simulink model "temp_gen_pch"  (Simulink 6.4)
settings: Solver=ode4  StartTime=0.0  StopTime=45  FixedStep=0.01  RelTol=1e-3
settings Model: Creator=oravec  LastModifiedBy=oravec
settings DataIOCC: LimitDataPoints=off  SignalLoggingName=sigsOut
settings OptimizationCC: InitFltsAndDblsToZero=off
settings DebuggingCC: SolverPrmCheckMsg=none  StrictBusMsg=None
settings HardwareCC: TargetHWDeviceType=32-bit Generic  TargetUnknown=on  ProdEqTarget=off

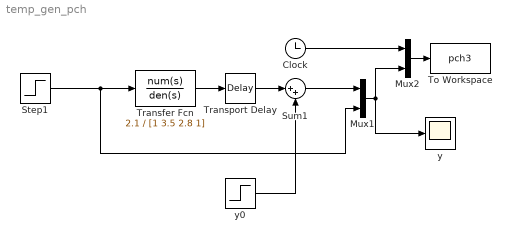
== system temp_gen_pch ==
  Clock : Clock
      settings: Decimation=10
  Mux1 : Mux  Inputs=2
  Mux2 : Mux  Inputs=2
  Step1 : Step  Time=0  Before=-1  After=2  SampleTime=0
  Sum1 : Sum  Inputs=|++
  To Workspace : ToWorkspace  VariableName=pch3  SampleTime=-1  SaveFormat=Array
  Transfer Fcn : TransferFcn  Numerator=2.1  Denominator=[1 3.5 2.8 1]
  Transport Delay : TransportDelay  DelayTime=0.3
  y : Scope
      settings: SaveName=ScopeData2
  y0 : Step  Time=0  After=3  SampleTime=0
  wires:
  Transfer Fcn/1 -> Transport Delay/1
  Mux1/1 -> y/1, Mux2/2
  Transport Delay/1 -> Sum1/1
  y0/1 -> Sum1/2
  Mux2/1 -> To Workspace/1
  Sum1/1 -> Mux1/1
  Clock/1 -> Mux2/1
  Step1/1 -> Transfer Fcn/1, Mux1/2
